simulink model "IBD"  (R2023a)
settings: Solver=VariableStepAuto  StartTime=0.0  StopTime=10.0  RelTol=1e-3
settings Model: Creator=woute  LastModifiedBy=woute

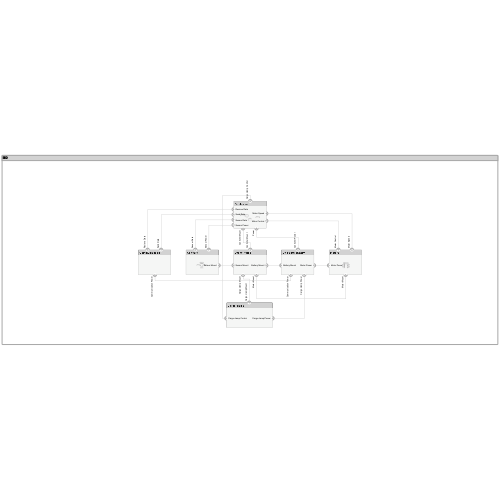
[thumbnail: Simulink's stored preview of the top-level diagram]
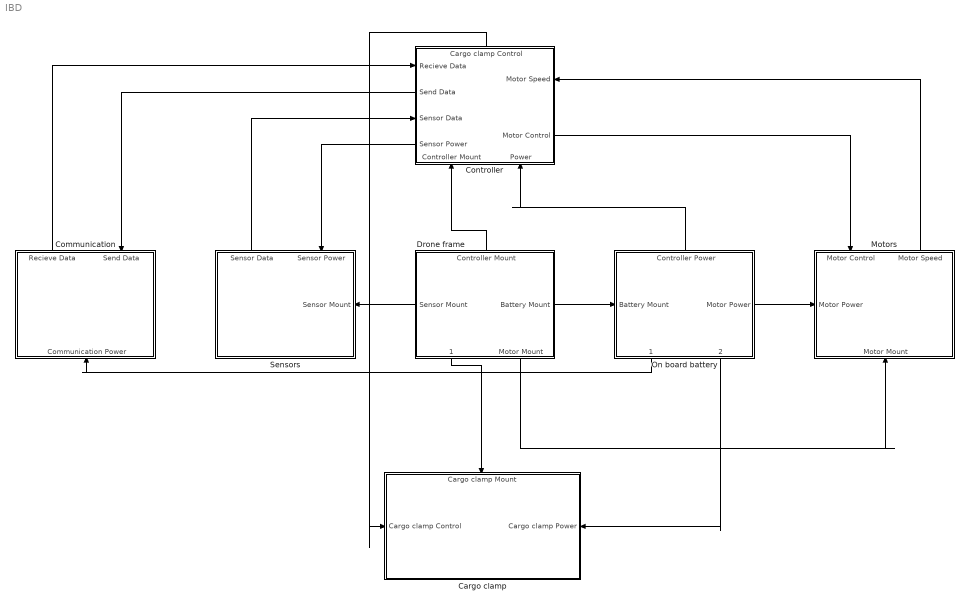
== system IBD ==
  Cargo clamp : Subsystem
      settings: PortSchema="{\"entries\":[{\"content\":{\"headerSize\":26,\"margin\":15,\"minimumSpacing\":25,\"sides\":[{\"content\":{\"connectorIds\":[\"In1\"]},\"type\":\"ConnectorPlacement.EquallySpacedRectSide\",\"uuid\":\"da0cf2bc-e0e5-43db-a533-396b99cf1bc7\"},{\"content\":{\"connectorIds\":[\"In2\"],\"side\":\"RIGHT\"},\"type\":\"ConnectorPlacement.EquallySpacedRectSide\",\"uuid\":\"a0b93c34-4dc2-4256-ba92-0f05a4d13f4f\"},{\"content\":{\"connectorIds\":[\"In3\"],\"side\":\"TOP\"},\"type\":\"ConnectorPlacement.EquallySpacedRectSide\",\"uuid\":\"6ebca4ef-ccb9-4ab5-864f-cbc834acd4e1\"}]},\"type\":\"ConnectorPlacement.EquallySpacedConnector\",\"uuid\":\"2b7ee882-fe9a-43a5-8f74-89585b316824\"}],\"packageUris\":[\"http://schema.mathworks.com/mf0/Connector/R2020b\"],\"version\":\"1.0\"}"
  Communication : Subsystem
      settings: PortSchema="{\"entries\":[{\"content\":{\"headerSize\":26,\"margin\":15,\"minimumSpacing\":25,\"sides\":[{\"content\":{},\"type\":\"ConnectorPlacement.EquallySpacedRectSide\",\"uuid\":\"da0cf2bc-e0e5-43db-a533-396b99cf1bc7\"},{\"content\":{\"side\":\"RIGHT\"},\"type\":\"ConnectorPlacement.EquallySpacedRectSide\",\"uuid\":\"a0b93c34-4dc2-4256-ba92-0f05a4d13f4f\"},{\"content\":{\"connectorIds\":[\"Out1\",\"In2\"],\"side\":\"TOP\"},\"type\":\"ConnectorPlacement.EquallySpacedRectSide\",\"uuid\":\"6ebca4ef-ccb9-4ab5-864f-cbc834acd4e1\"},{\"content\":{\"connectorIds\":[\"In1\"],\"side\":\"BOTTOM\"},\"type\":\"ConnectorPlacement.EquallySpacedRectSide\",\"uuid\":\"1374c768-d183-49b7-a66a-8b95b6ecd3ed\"}]},\"type\":\"ConnectorPlacement.EquallySpacedConnector\",\"uuid\":\"2b7ee882-fe9a-43a5-8f74-89585b316824\"}],\"packageUris\":[\"http://schema.mathworks.com/mf0/Connector/R2020b\"],\"version\":\"1.0\"}"
  Controller : Subsystem
      settings: PortSchema="{\"entries\":[{\"content\":{\"headerSize\":26,\"margin\":15,\"minimumSpacing\":25,\"sides\":[{\"content\":{\"connectorIds\":[\"In2\",\"Out1\",\"In3\",\"Out3\"]},\"type\":\"ConnectorPlacement.EquallySpacedRectSide\",\"uuid\":\"da0cf2bc-e0e5-43db-a533-396b99cf1bc7\"},{\"content\":{\"connectorIds\":[\"In1\",\"Out2\"],\"side\":\"RIGHT\"},\"type\":\"ConnectorPlacement.EquallySpacedRectSide\",\"uuid\":\"a0b93c34-4dc2-4256-ba92-0f05a4d13f4f\"},{\"content\":{\"connectorIds\":[\"Out4\"],\"side\":\"TOP\"},\"type\":\"ConnectorPlacement.EquallySpacedRectSide\",\"uuid\":\"6ebca4ef-ccb9-4ab5-864f-cbc834acd4e1\"},{\"content\":{\"connectorIds\":[\"In4\",\"In5\"],\"side\":\"BOTTOM\"},\"type\":\"ConnectorPlacement.EquallySpacedRectSide\",\"uuid\":\"e70a3738-18ab-432b-b547-bc9088a076a5\"}]},\"type\":\"ConnectorPlacement.EquallySpacedConnector\",\"uuid\":\"2b7ee882-fe9a-43a5-8f74-89585b316824\"}],\"packageUris\":[\"http://schema.mathworks.com/mf0/Connector/R2020b\"],\"version\":\"1.0\"}"
  Drone frame : Subsystem
      settings: PortSchema="{\"entries\":[{\"content\":{\"headerSize\":26,\"margin\":15,\"minimumSpacing\":25,\"sides\":[{\"content\":{\"connectorIds\":[\"Out5\"]},\"type\":\"ConnectorPlacement.EquallySpacedRectSide\",\"uuid\":\"da0cf2bc-e0e5-43db-a533-396b99cf1bc7\"},{\"content\":{\"connectorIds\":[\"Out4\"],\"side\":\"RIGHT\"},\"type\":\"ConnectorPlacement.EquallySpacedRectSide\",\"uuid\":\"a0b93c34-4dc2-4256-ba92-0f05a4d13f4f\"},{\"content\":{\"connectorIds\":[\"Out3\"],\"side\":\"TOP\"},\"type\":\"ConnectorPlacement.EquallySpacedRectSide\",\"uuid\":\"6ebca4ef-ccb9-4ab5-864f-cbc834acd4e1\"},{\"content\":{\"connectorIds\":[\"Out1\",\"Out2\"],\"side\":\"BOTTOM\"},\"type\":\"ConnectorPlacement.EquallySpacedRectSide\",\"uuid\":\"4cad4506-a5db-4877-9d67-f341f6b35e14\"}]},\"type\":\"ConnectorPlacement.EquallySpacedConnector\",\"uuid\":\"2b7ee882-fe9a-43a5-8f74-89585b316824\"}],\"packageUris\":[\"http://schema.mathworks.com/mf0/Connector/R2020b\"],\"version\":\"1.0\"}"
  Motors : Subsystem
      settings: PortSchema="{\"entries\":[{\"content\":{\"headerSize\":26,\"margin\":15,\"minimumSpacing\":25,\"sides\":[{\"content\":{\"connectorIds\":[\"In2\"]},\"type\":\"ConnectorPlacement.EquallySpacedRectSide\",\"uuid\":\"da0cf2bc-e0e5-43db-a533-396b99cf1bc7\"},{\"content\":{\"side\":\"RIGHT\"},\"type\":\"ConnectorPlacement.EquallySpacedRectSide\",\"uuid\":\"a0b93c34-4dc2-4256-ba92-0f05a4d13f4f\"},{\"content\":{\"connectorIds\":[\"In1\",\"Out1\"],\"side\":\"TOP\"},\"type\":\"ConnectorPlacement.EquallySpacedRectSide\",\"uuid\":\"6ebca4ef-ccb9-4ab5-864f-cbc834acd4e1\"},{\"content\":{\"connectorIds\":[\"In3\"],\"side\":\"BOTTOM\"},\"type\":\"ConnectorPlacement.EquallySpacedRectSide\",\"uuid\":\"1374c768-d183-49b7-a66a-8b95b6ecd3ed\"}]},\"type\":\"ConnectorPlacement.EquallySpacedConnector\",\"uuid\":\"2b7ee882-fe9a-43a5-8f74-89585b316824\"}],\"packageUris\":[\"http://schema.mathworks.com/mf0/Connector/R2020b\"],\"version\":\"1.0\"}"
  On board battery : Subsystem
      settings: PortSchema="{\"entries\":[{\"content\":{\"headerSize\":26,\"margin\":15,\"minimumSpacing\":25,\"sides\":[{\"content\":{\"connectorIds\":[\"In1\"]},\"type\":\"ConnectorPlacement.EquallySpacedRectSide\",\"uuid\":\"da0cf2bc-e0e5-43db-a533-396b99cf1bc7\"},{\"content\":{\"connectorIds\":[\"Out3\"],\"side\":\"RIGHT\"},\"type\":\"ConnectorPlacement.EquallySpacedRectSide\",\"uuid\":\"a0b93c34-4dc2-4256-ba92-0f05a4d13f4f\"},{\"content\":{\"connectorIds\":[\"Out4\"],\"side\":\"TOP\"},\"type\":\"ConnectorPlacement.EquallySpacedRectSide\",\"uuid\":\"6ebca4ef-ccb9-4ab5-864f-cbc834acd4e1\"},{\"content\":{\"connectorIds\":[\"Out1\",\"Out2\"],\"side\":\"BOTTOM\"},\"type\":\"ConnectorPlacement.EquallySpacedRectSide\",\"uuid\":\"3e1d13d2-d0a6-4e10-b525-4004a1834e49\"}]},\"type\":\"ConnectorPlacement.EquallySpacedConnector\",\"uuid\":\"2b7ee882-fe9a-43a5-8f74-89585b316824\"}],\"packageUris\":[\"http://schema.mathworks.com/mf0/Connector/R2020b\"],\"version\":\"1.0\"}"
  Sensors : Subsystem
      settings: PortSchema="{\"entries\":[{\"content\":{\"headerSize\":26,\"margin\":15,\"minimumSpacing\":25,\"sides\":[{\"content\":{},\"type\":\"ConnectorPlacement.EquallySpacedRectSide\",\"uuid\":\"da0cf2bc-e0e5-43db-a533-396b99cf1bc7\"},{\"content\":{\"connectorIds\":[\"In2\"],\"side\":\"RIGHT\"},\"type\":\"ConnectorPlacement.EquallySpacedRectSide\",\"uuid\":\"a0b93c34-4dc2-4256-ba92-0f05a4d13f4f\"},{\"content\":{\"connectorIds\":[\"Out1\",\"In1\"],\"side\":\"TOP\"},\"type\":\"ConnectorPlacement.EquallySpacedRectSide\",\"uuid\":\"6ebca4ef-ccb9-4ab5-864f-cbc834acd4e1\"}]},\"type\":\"ConnectorPlacement.EquallySpacedConnector\",\"uuid\":\"2b7ee882-fe9a-43a5-8f74-89585b316824\"}],\"packageUris\":[\"http://schema.mathworks.com/mf0/Connector/R2020b\"],\"version\":\"1.0\"}"
  wires:
  Controller/2(Motor Control) -> Motors/1(Motor Control)
  On board battery/3(Motor Power) -> Motors/2(Motor Power)
  Drone frame/1(Cargo clamp Mount) -> Cargo clamp/3(Cargo clamp Mount)
  Controller/4(Cargo clamp Control) -> Cargo clamp/1(Cargo clamp Control)
  Communication/1(Recieve Data) -> Controller/2(Recieve Data)
  Motors/1(Motor Speed) -> Controller/1(Motor Speed)
  Drone frame/5(Sensor Mount) -> Sensors/2(Sensor Mount)
  Controller/1(Send Data) -> Communication/2(Send Data)
  On board battery/1(Communication Power) -> Communication/1(Communication Power)
  On board battery/2(Cargo clamp Power) -> Cargo clamp/2(Cargo clamp Power)
  Drone frame/2(Motor Mount) -> Motors/3(Motor Mount)
  Drone frame/3(Controller Mount) -> Controller/4(Controller Mount)
  On board battery/4(Controller Power) -> Controller/5(Power)
  Controller/3(Sensor Power) -> Sensors/1(Sensor Power)
  Sensors/1(Sensor Data) -> Controller/3(Sensor Data)
  Drone frame/4(Battery Mount) -> On board battery/1(Battery Mount)

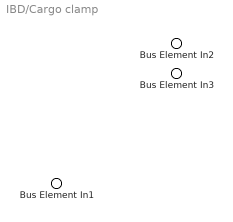
== system IBD/Cargo clamp ==
  Bus Element In3 : Inport  PortName=Cargo clamp Control
  Bus Element In2 : Inport  Port=2  PortName=Cargo clamp Power
  Bus Element In1 : Inport  Port=3  PortName=Cargo clamp Mount

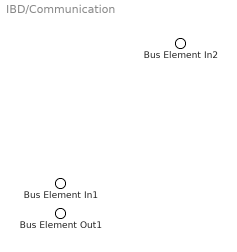
== system IBD/Communication ==
  Bus Element In2 : Inport  PortName=Communication Power
  Bus Element In1 : Inport  Port=2  PortName=Send Data
  Bus Element Out1 : Outport  PortName=Recieve Data

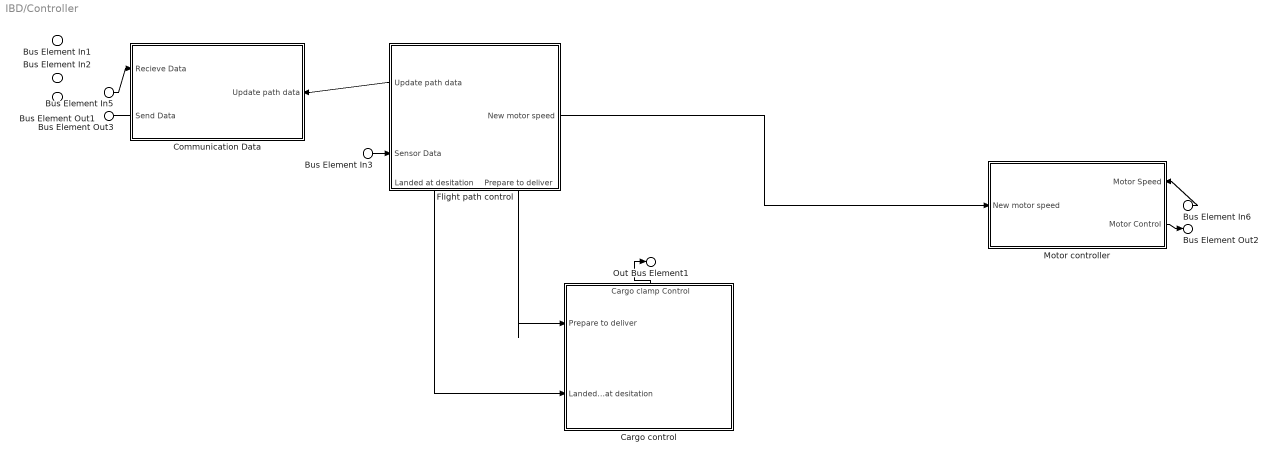
== system IBD/Controller ==
  Bus Element In6 : Inport  PortName=Motor Speed
  Bus Element In5 : Inport  Port=2  PortName=Recieve Data
  Bus Element In3 : Inport  Port=3  PortName=Sensor Data
  Bus Element In1 : Inport  Port=4  PortName=Controller Mount
  Bus Element In2 : Inport  Port=5  PortName=Power
  Cargo control : Subsystem
      settings: PortSchema="{\"entries\":[{\"content\":{\"headerSize\":26,\"margin\":15,\"minimumSpacing\":25,\"sides\":[{\"content\":{\"connectorIds\":[\"In1\",\"In2\"]},\"type\":\"ConnectorPlacement.EquallySpacedRectSide\",\"uuid\":\"47abfa5f-2965-4884-af59-19e27a1fecc5\"},{\"content\":{\"side\":\"RIGHT\"},\"type\":\"ConnectorPlacement.EquallySpacedRectSide\",\"uuid\":\"258bf353-9708-4540-ba01-9a9d579047ae\"},{\"content\":{\"connectorIds\":[\"Out1\"],\"side\":\"TOP\"},\"type\":\"ConnectorPlacement.EquallySpacedRectSide\",\"uuid\":\"d7a7d3fb-c4c1-4c02-9f4a-88d006008406\"}]},\"type\":\"ConnectorPlacement.EquallySpacedConnector\",\"uuid\":\"3695f6c5-486f-42c8-b025-c0248a78a2e8\"}],\"packageUris\":[\"http://schema.mathworks.com/mf0/Connector/R2020b\"],\"version\":\"1.0\"}"
  Communication Data : Subsystem
      settings: PortSchema="{\"entries\":[{\"content\":{\"headerSize\":26,\"margin\":15,\"minimumSpacing\":25,\"sides\":[{\"content\":{\"connectorIds\":[\"In2\",\"Out1\"]},\"type\":\"ConnectorPlacement.EquallySpacedRectSide\",\"uuid\":\"47abfa5f-2965-4884-af59-19e27a1fecc5\"},{\"content\":{\"connectorIds\":[\"In1\"],\"side\":\"RIGHT\"},\"type\":\"ConnectorPlacement.EquallySpacedRectSide\",\"uuid\":\"258bf353-9708-4540-ba01-9a9d579047ae\"},{\"content\":{\"side\":\"TOP\"},\"type\":\"ConnectorPlacement.EquallySpacedRectSide\",\"uuid\":\"d7a7d3fb-c4c1-4c02-9f4a-88d006008406\"}]},\"type\":\"ConnectorPlacement.EquallySpacedConnector\",\"uuid\":\"3695f6c5-486f-42c8-b025-c0248a78a2e8\"}],\"packageUris\":[\"http://schema.mathworks.com/mf0/Connector/R2020b\"],\"version\":\"1.0\"}"
  Flight path control : Subsystem
      settings: PortSchema="{\"entries\":[{\"content\":{\"headerSize\":26,\"margin\":15,\"minimumSpacing\":25,\"sides\":[{\"content\":{\"connectorIds\":[\"Out4\",\"In1\"]},\"type\":\"ConnectorPlacement.EquallySpacedRectSide\",\"uuid\":\"47abfa5f-2965-4884-af59-19e27a1fecc5\"},{\"content\":{\"connectorIds\":[\"Out3\"],\"side\":\"RIGHT\"},\"type\":\"ConnectorPlacement.EquallySpacedRectSide\",\"uuid\":\"258bf353-9708-4540-ba01-9a9d579047ae\"},{\"content\":{\"side\":\"TOP\"},\"type\":\"ConnectorPlacement.EquallySpacedRectSide\",\"uuid\":\"d7a7d3fb-c4c1-4c02-9f4a-88d006008406\"},{\"content\":{\"connectorIds\":[\"Out1\",\"Out2\"],\"side\":\"BOTTOM\"},\"type\":\"ConnectorPlacement.EquallySpacedRectSide\",\"uuid\":\"f22d4cbb-a1fb-4732-9001-824522f19399\"}]},\"type\":\"ConnectorPlacement.EquallySpacedConnector\",\"uuid\":\"3695f6c5-486f-42c8-b025-c0248a78a2e8\"}],\"packageUris\":[\"http://schema.mathworks.com/mf0/Connector/R2020b\"],\"version\":\"1.0\"}"
  Motor controller : Subsystem
      settings: PortSchema="{\"entries\":[{\"content\":{\"headerSize\":26,\"margin\":15,\"minimumSpacing\":25,\"sides\":[{\"content\":{\"connectorIds\":[\"In1\"]},\"type\":\"ConnectorPlacement.EquallySpacedRectSide\",\"uuid\":\"47abfa5f-2965-4884-af59-19e27a1fecc5\"},{\"content\":{\"connectorIds\":[\"In2\",\"Out1\"],\"side\":\"RIGHT\"},\"type\":\"ConnectorPlacement.EquallySpacedRectSide\",\"uuid\":\"258bf353-9708-4540-ba01-9a9d579047ae\"},{\"content\":{\"side\":\"TOP\"},\"type\":\"ConnectorPlacement.EquallySpacedRectSide\",\"uuid\":\"d7a7d3fb-c4c1-4c02-9f4a-88d006008406\"}]},\"type\":\"ConnectorPlacement.EquallySpacedConnector\",\"uuid\":\"3695f6c5-486f-42c8-b025-c0248a78a2e8\"}],\"packageUris\":[\"http://schema.mathworks.com/mf0/Connector/R2020b\"],\"version\":\"1.0\"}"
  Bus Element Out3 : Outport  PortName=Send Data
  Bus Element Out2 : Outport  Port=2  PortName=Motor Control
  Bus Element Out1 : Outport  Port=3  PortName=Sensor Power
  Out Bus Element1 : Outport  Port=4  PortName=Cargo clamp Control
  wires:
  Motor controller/1(Motor Control) -> Bus Element Out2/1
  Bus Element In6/1 -> Motor controller/2(Motor Speed)
  Bus Element In5/1 -> Communication Data/2(Recieve Data)
  Communication Data/1(Send Data) -> Bus Element Out3/1
  Bus Element In3/1 -> Flight path control/1(Sensor Data)
  Flight path control/4(Update path data) -> Communication Data/1(Update path data)
  Flight path control/3(New motor speed) -> Motor controller/1(New motor speed)
  Flight path control/1(Landed at desitation) -> Cargo control/2(Landed at desitation)
  Cargo control/1(Cargo clamp Control) -> Out Bus Element1/1
  Flight path control/2(Prepare to deliver) -> Cargo control/1(Prepare to deliver)

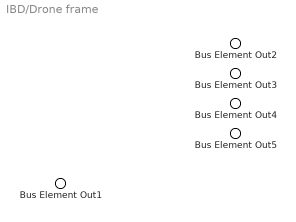
== system IBD/Drone frame ==
  Bus Element Out4 : Outport  PortName=Cargo clamp Mount
  Bus Element Out5 : Outport  Port=2  PortName=Motor Mount
  Bus Element Out3 : Outport  Port=3  PortName=Controller Mount
  Bus Element Out2 : Outport  Port=4  PortName=Battery Mount
  Bus Element Out1 : Outport  Port=5  PortName=Sensor Mount

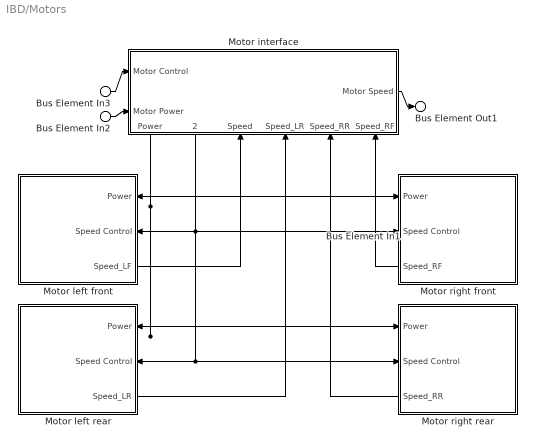
== system IBD/Motors ==
  Bus Element In3 : Inport  PortName=Motor Control
  Bus Element In2 : Inport  Port=2  PortName=Motor Power
  Bus Element In1 : Inport  Port=3  PortName=Motor Mount
  Motor interface : Subsystem
      settings: PortSchema="{\"entries\":[{\"content\":{\"headerSize\":26,\"margin\":15,\"minimumSpacing\":25,\"sides\":[{\"content\":{\"connectorIds\":[\"In5\",\"In6\"]},\"type\":\"ConnectorPlacement.EquallySpacedRectSide\",\"uuid\":\"47abfa5f-2965-4884-af59-19e27a1fecc5\"},{\"content\":{\"connectorIds\":[\"Out3\"],\"side\":\"RIGHT\"},\"type\":\"ConnectorPlacement.EquallySpacedRectSide\",\"uuid\":\"258bf353-9708-4540-ba01-9a9d579047ae\"},{\"content\":{\"side\":\"TOP\"},\"type\":\"ConnectorPlacement.EquallySpacedRectSide\",\"uuid\":\"d7a7d3fb-c4c1-4c02-9f4a-88d006008406\"},{\"content\":{\"connectorIds\":[\"Out1\",\"Out2\",\"In1\",\"In2\",\"In3\",\"In4\"],\"side\":\"BOTTOM\"},\"type\":\"ConnectorPlacement.EquallySpacedRectSide\",\"uuid\":\"016b631c-414c-488e-95c2-b28873815a5f\"}]},\"type\":\"ConnectorPlacement.EquallySpacedConnector\",\"uuid\":\"3695f6c5-486f-42c8-b025-c0248a78a2e8\"}],\"packageUris\":[\"http://schema.mathworks.com/mf0/Connector/R2020b\"],\"version\":\"1.0\"}"
  Motor left front : Subsystem
      settings: PortSchema="{\"entries\":[{\"content\":{\"headerSize\":26,\"margin\":15,\"minimumSpacing\":25,\"sides\":[{\"content\":{},\"type\":\"ConnectorPlacement.EquallySpacedRectSide\",\"uuid\":\"47abfa5f-2965-4884-af59-19e27a1fecc5\"},{\"content\":{\"connectorIds\":[\"In1\",\"In2\",\"Out1\"],\"side\":\"RIGHT\"},\"type\":\"ConnectorPlacement.EquallySpacedRectSide\",\"uuid\":\"258bf353-9708-4540-ba01-9a9d579047ae\"},{\"content\":{\"side\":\"TOP\"},\"type\":\"ConnectorPlacement.EquallySpacedRectSide\",\"uuid\":\"d7a7d3fb-c4c1-4c02-9f4a-88d006008406\"}]},\"type\":\"ConnectorPlacement.EquallySpacedConnector\",\"uuid\":\"3695f6c5-486f-42c8-b025-c0248a78a2e8\"}],\"packageUris\":[\"http://schema.mathworks.com/mf0/Connector/R2020b\"],\"version\":\"1.0\"}"
  Motor left rear : Subsystem
      settings: PortSchema="{\"entries\":[{\"content\":{\"headerSize\":26,\"margin\":15,\"minimumSpacing\":25,\"sides\":[{\"content\":{},\"type\":\"ConnectorPlacement.EquallySpacedRectSide\",\"uuid\":\"47abfa5f-2965-4884-af59-19e27a1fecc5\"},{\"content\":{\"connectorIds\":[\"In1\",\"In2\",\"Out1\"],\"side\":\"RIGHT\"},\"type\":\"ConnectorPlacement.EquallySpacedRectSide\",\"uuid\":\"258bf353-9708-4540-ba01-9a9d579047ae\"},{\"content\":{\"side\":\"TOP\"},\"type\":\"ConnectorPlacement.EquallySpacedRectSide\",\"uuid\":\"d7a7d3fb-c4c1-4c02-9f4a-88d006008406\"}]},\"type\":\"ConnectorPlacement.EquallySpacedConnector\",\"uuid\":\"3695f6c5-486f-42c8-b025-c0248a78a2e8\"}],\"packageUris\":[\"http://schema.mathworks.com/mf0/Connector/R2020b\"],\"version\":\"1.0\"}"
  Motor right front : Subsystem
      settings: PortSchema="{\"entries\":[{\"content\":{\"headerSize\":26,\"margin\":15,\"minimumSpacing\":25,\"sides\":[{\"content\":{\"connectorIds\":[\"In1\",\"In2\",\"Out1\"]},\"type\":\"ConnectorPlacement.EquallySpacedRectSide\",\"uuid\":\"47abfa5f-2965-4884-af59-19e27a1fecc5\"},{\"content\":{\"side\":\"RIGHT\"},\"type\":\"ConnectorPlacement.EquallySpacedRectSide\",\"uuid\":\"258bf353-9708-4540-ba01-9a9d579047ae\"},{\"content\":{\"side\":\"TOP\"},\"type\":\"ConnectorPlacement.EquallySpacedRectSide\",\"uuid\":\"d7a7d3fb-c4c1-4c02-9f4a-88d006008406\"}]},\"type\":\"ConnectorPlacement.EquallySpacedConnector\",\"uuid\":\"3695f6c5-486f-42c8-b025-c0248a78a2e8\"}],\"packageUris\":[\"http://schema.mathworks.com/mf0/Connector/R2020b\"],\"version\":\"1.0\"}"
  Motor right rear : Subsystem
      settings: PortSchema="{\"entries\":[{\"content\":{\"headerSize\":26,\"margin\":15,\"minimumSpacing\":25,\"sides\":[{\"content\":{\"connectorIds\":[\"In1\",\"In2\",\"Out1\"]},\"type\":\"ConnectorPlacement.EquallySpacedRectSide\",\"uuid\":\"47abfa5f-2965-4884-af59-19e27a1fecc5\"},{\"content\":{\"side\":\"RIGHT\"},\"type\":\"ConnectorPlacement.EquallySpacedRectSide\",\"uuid\":\"258bf353-9708-4540-ba01-9a9d579047ae\"},{\"content\":{\"side\":\"TOP\"},\"type\":\"ConnectorPlacement.EquallySpacedRectSide\",\"uuid\":\"d7a7d3fb-c4c1-4c02-9f4a-88d006008406\"}]},\"type\":\"ConnectorPlacement.EquallySpacedConnector\",\"uuid\":\"3695f6c5-486f-42c8-b025-c0248a78a2e8\"}],\"packageUris\":[\"http://schema.mathworks.com/mf0/Connector/R2020b\"],\"version\":\"1.0\"}"
  Bus Element Out1 : Outport  PortName=Motor Speed
  wires:
  Bus Element In3/1 -> Motor interface/5(Motor Control)
  Motor interface/3(Motor Speed) -> Bus Element Out1/1
  Bus Element In2/1 -> Motor interface/6(Motor Power)
  Motor interface/1(Power) -> Motor right rear/1(Power), Motor left rear/1(Power), Motor right front/1(Power), Motor left front/1(Power)
  Motor interface/2(Speed Control) -> Motor left rear/2(Speed Control), Motor right rear/2(Speed Control), Motor right front/2(Speed Control), Motor left front/2(Speed Control)
  Motor left front/1(Speed_LF) -> Motor interface/1(Speed)
  Motor right front/1(Speed_RF) -> Motor interface/4(Speed_RF)
  Motor right rear/1(Speed_RR) -> Motor interface/3(Speed_RR)
  Motor left rear/1(Speed_LR) -> Motor interface/2(Speed_LR)

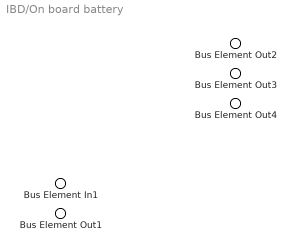
== system IBD/On board battery ==
  Bus Element In1 : Inport  PortName=Battery Mount
  Bus Element Out4 : Outport  PortName=Communication Power
  Bus Element Out3 : Outport  Port=2  PortName=Cargo clamp Power
  Bus Element Out2 : Outport  Port=3  PortName=Motor Power
  Bus Element Out1 : Outport  Port=4  PortName=Controller Power

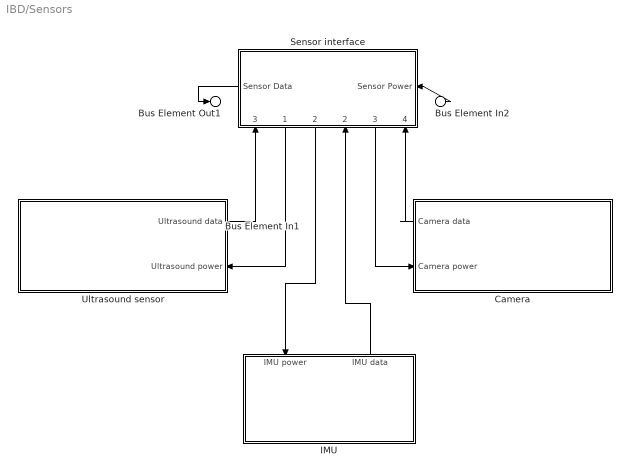
== system IBD/Sensors ==
  Bus Element In2 : Inport  PortName=Sensor Power
  Bus Element In1 : Inport  Port=2  PortName=Sensor Mount
  Camera : Subsystem
      settings: PortSchema="{\"entries\":[{\"content\":{\"headerSize\":26,\"margin\":15,\"minimumSpacing\":25,\"sides\":[{\"content\":{\"connectorIds\":[\"Out1\",\"In1\"]},\"type\":\"ConnectorPlacement.EquallySpacedRectSide\",\"uuid\":\"47abfa5f-2965-4884-af59-19e27a1fecc5\"},{\"content\":{\"side\":\"RIGHT\"},\"type\":\"ConnectorPlacement.EquallySpacedRectSide\",\"uuid\":\"258bf353-9708-4540-ba01-9a9d579047ae\"},{\"content\":{\"side\":\"TOP\"},\"type\":\"ConnectorPlacement.EquallySpacedRectSide\",\"uuid\":\"d7a7d3fb-c4c1-4c02-9f4a-88d006008406\"}]},\"type\":\"ConnectorPlacement.EquallySpacedConnector\",\"uuid\":\"3695f6c5-486f-42c8-b025-c0248a78a2e8\"}],\"packageUris\":[\"http://schema.mathworks.com/mf0/Connector/R2020b\"],\"version\":\"1.0\"}"
  IMU : Subsystem
      settings: PortSchema="{\"entries\":[{\"content\":{\"headerSize\":26,\"margin\":15,\"minimumSpacing\":25,\"sides\":[{\"content\":{},\"type\":\"ConnectorPlacement.EquallySpacedRectSide\",\"uuid\":\"47abfa5f-2965-4884-af59-19e27a1fecc5\"},{\"content\":{\"side\":\"RIGHT\"},\"type\":\"ConnectorPlacement.EquallySpacedRectSide\",\"uuid\":\"258bf353-9708-4540-ba01-9a9d579047ae\"},{\"content\":{\"connectorIds\":[\"In1\",\"Out1\"],\"side\":\"TOP\"},\"type\":\"ConnectorPlacement.EquallySpacedRectSide\",\"uuid\":\"d7a7d3fb-c4c1-4c02-9f4a-88d006008406\"}]},\"type\":\"ConnectorPlacement.EquallySpacedConnector\",\"uuid\":\"3695f6c5-486f-42c8-b025-c0248a78a2e8\"}],\"packageUris\":[\"http://schema.mathworks.com/mf0/Connector/R2020b\"],\"version\":\"1.0\"}"
  Sensor interface : Subsystem
      settings: PortSchema="{\"entries\":[{\"content\":{\"headerSize\":26,\"margin\":15,\"minimumSpacing\":25,\"sides\":[{\"content\":{\"connectorIds\":[\"Out4\"]},\"type\":\"ConnectorPlacement.EquallySpacedRectSide\",\"uuid\":\"47abfa5f-2965-4884-af59-19e27a1fecc5\"},{\"content\":{\"connectorIds\":[\"In1\"],\"side\":\"RIGHT\"},\"type\":\"ConnectorPlacement.EquallySpacedRectSide\",\"uuid\":\"258bf353-9708-4540-ba01-9a9d579047ae\"},{\"content\":{\"side\":\"TOP\"},\"type\":\"ConnectorPlacement.EquallySpacedRectSide\",\"uuid\":\"d7a7d3fb-c4c1-4c02-9f4a-88d006008406\"},{\"content\":{\"connectorIds\":[\"In3\",\"Out1\",\"Out2\",\"In2\",\"Out3\",\"In4\"],\"side\":\"BOTTOM\"},\"type\":\"ConnectorPlacement.EquallySpacedRectSide\",\"uuid\":\"f9931c82-3cac-403f-a246-b2b88de51d1b\"}]},\"type\":\"ConnectorPlacement.EquallySpacedConnector\",\"uuid\":\"3695f6c5-486f-42c8-b025-c0248a78a2e8\"}],\"packageUris\":[\"http://schema.mathworks.com/mf0/Connector/R2020b\"],\"version\":\"1.0\"}"
  Ultrasound sensor : Subsystem
      settings: PortSchema="{\"entries\":[{\"content\":{\"headerSize\":26,\"margin\":15,\"minimumSpacing\":25,\"sides\":[{\"content\":{},\"type\":\"ConnectorPlacement.EquallySpacedRectSide\",\"uuid\":\"47abfa5f-2965-4884-af59-19e27a1fecc5\"},{\"content\":{\"connectorIds\":[\"Out1\",\"In1\"],\"side\":\"RIGHT\"},\"type\":\"ConnectorPlacement.EquallySpacedRectSide\",\"uuid\":\"258bf353-9708-4540-ba01-9a9d579047ae\"},{\"content\":{\"side\":\"TOP\"},\"type\":\"ConnectorPlacement.EquallySpacedRectSide\",\"uuid\":\"d7a7d3fb-c4c1-4c02-9f4a-88d006008406\"}]},\"type\":\"ConnectorPlacement.EquallySpacedConnector\",\"uuid\":\"3695f6c5-486f-42c8-b025-c0248a78a2e8\"}],\"packageUris\":[\"http://schema.mathworks.com/mf0/Connector/R2020b\"],\"version\":\"1.0\"}"
  Bus Element Out1 : Outport  PortName=Sensor Data
  wires:
  Ultrasound sensor/1(Ultrasound data) -> Sensor interface/3(Ultrasound data)
  Camera/1(Camera data) -> Sensor interface/4(Camera data)
  Sensor interface/4(Sensor Data) -> Bus Element Out1/1
  Bus Element In2/1 -> Sensor interface/1(Sensor Power)
  Sensor interface/1(Ultrasound power) -> Ultrasound sensor/1(Ultrasound power)
  Sensor interface/3(Camera power) -> Camera/1(Camera power)
  Sensor interface/2(IMU power) -> IMU/1(IMU power)
  IMU/1(IMU data) -> Sensor interface/2(IMU data)

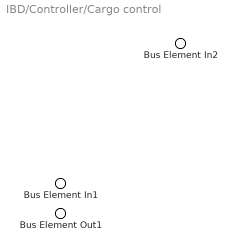
== system IBD/Controller/Cargo control ==
  Bus Element In2 : Inport  PortName=Prepare to deliver
  Bus Element In1 : Inport  Port=2  PortName=Landed at desitation
  Bus Element Out1 : Outport  PortName=Cargo clamp Control

== system IBD/Controller/Communication Data ==
  Bus Element In2 : Inport  PortName=Update path data
  Bus Element In1 : Inport  Port=2  PortName=Recieve Data
  Bus Element Out1 : Outport  PortName=Send Data

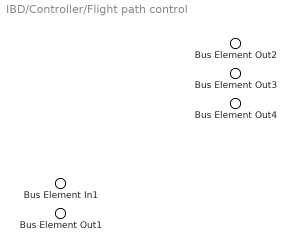
== system IBD/Controller/Flight path control ==
  Bus Element In1 : Inport  PortName=Sensor Data
  Bus Element Out3 : Outport  PortName=Landed at desitation
  Bus Element Out4 : Outport  Port=2  PortName=Prepare to deliver
  Bus Element Out2 : Outport  Port=3  PortName=New motor speed
  Bus Element Out1 : Outport  Port=4  PortName=Update path data

== system IBD/Controller/Motor controller ==
  Bus Element In2 : Inport  PortName=New motor speed
  Bus Element In1 : Inport  Port=2  PortName=Motor Speed
  Bus Element Out1 : Outport  PortName=Motor Control

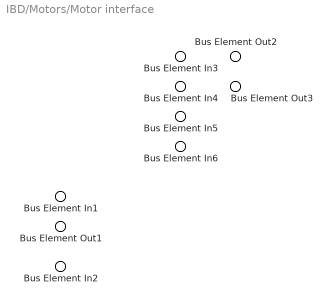
== system IBD/Motors/Motor interface ==
  Bus Element In3 : Inport  PortName=Speed
  Bus Element In6 : Inport  Port=2  PortName=Speed_LR
  Bus Element In5 : Inport  Port=3  PortName=Speed_RR
  Bus Element In4 : Inport  Port=4  PortName=Speed_RF
  Bus Element In1 : Inport  Port=5  PortName=Motor Control
  Bus Element In2 : Inport  Port=6  PortName=Motor Power
  Bus Element Out2 : Outport  PortName=Power
  Bus Element Out3 : Outport  Port=2  PortName=Speed Control
  Bus Element Out1 : Outport  Port=3  PortName=Motor Speed

== system IBD/Motors/Motor left front ==
  In Bus Element1 : Inport  PortName=Power
  Bus Element In2 : Inport  Port=2  PortName=Speed Control
  Bus Element Out1 : Outport  PortName=Speed_LF

== system IBD/Motors/Motor left rear ==
  Bus Element In1 : Inport  PortName=Power
  Bus Element In2 : Inport  Port=2  PortName=Speed Control
  Bus Element Out1 : Outport  PortName=Speed_LR

== system IBD/Motors/Motor right front ==
  Bus Element In1 : Inport  PortName=Power
  Bus Element In2 : Inport  Port=2  PortName=Speed Control
  Bus Element Out1 : Outport  PortName=Speed_RF

== system IBD/Motors/Motor right rear ==
  Bus Element In1 : Inport  PortName=Power
  Bus Element In2 : Inport  Port=2  PortName=Speed Control
  Bus Element Out1 : Outport  PortName=Speed_RR

== system IBD/Sensors/Camera ==
  Bus Element In1 : Inport  PortName=Camera power
  Bus Element Out1 : Outport  PortName=Camera data

== system IBD/Sensors/IMU ==
  Bus Element In1 : Inport  PortName=IMU power
  Bus Element Out1 : Outport  PortName=IMU data

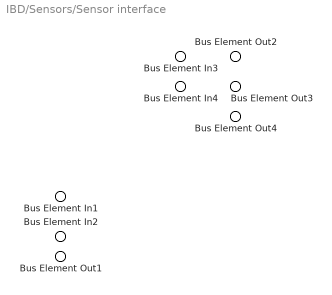
== system IBD/Sensors/Sensor interface ==
  Bus Element In3 : Inport  PortName=Sensor Power
  Bus Element In4 : Inport  Port=2  PortName=IMU data
  Bus Element In1 : Inport  Port=3  PortName=Ultrasound data
  Bus Element In2 : Inport  Port=4  PortName=Camera data
  Bus Element Out2 : Outport  PortName=Ultrasound power
  Bus Element Out4 : Outport  Port=2  PortName=IMU power
  Bus Element Out3 : Outport  Port=3  PortName=Camera power
  Bus Element Out1 : Outport  Port=4  PortName=Sensor Data

== system IBD/Sensors/Ultrasound sensor ==
  Bus Element In1 : Inport  PortName=Ultrasound power
  Bus Element Out1 : Outport  PortName=Ultrasound data
